simulink model "test44"  (R2015a)
settings: Solver=ode45  StartTime=0.0  StopTime=10.0  RelTol=1e-3
values from neighbouring files (symbols this model uses):
  Ac = A - B*K + L*C    [test3.m]    (also in test4.m; test5.m)
  Bc = -L    [test3.m]    (also in test4.m; test5.m)
  Cc = K    [test3.m]    (also in test4.m; test5.m)
  d1 = m0 + m1 + m2    (= 2.75)    [test3.m]    (also in test4.m; test5.m = 0.00498784618394)
  d2 = (m1/2 + m2) * l1    (= 0.5)    [test3.m]    (also in test4.m; test5.m = 0.00670234055869)
  d3 = m2 * l2/2    (= 0.28125)    [test3.m]    (also in test4.m; test5.m = 0.00902586221044)
  d4 = (m1/3 + m2) * l1^2    (= 0.229166666667)    [test3.m]    (also in test4.m)
  d5 = m2 * l1 * l2/2    (= 0.140625)    [test3.m]    (also in test4.m)
  d6 = m2 * l2^2/3    (= 0.140625)    [test3.m]    (also in test4.m)
  Dc = 0    [test3.m]    (also in test4.m; test5.m)
  f1 = (m1/2 + m2) * l1 * g    (= 4.9)    [test3.m]    (also in test4.m; test5.m = 0.66350669926)
  f2 = m2 * l2 *g/2    (= 2.75625)    [test3.m]    (also in test4.m; test5.m = 0.891162386564)
  r = 0    [test2.m]    (also in test3.m; test4.m; test5.m)
settings Model: Creator=joseg  LastModifiedBy=joseg

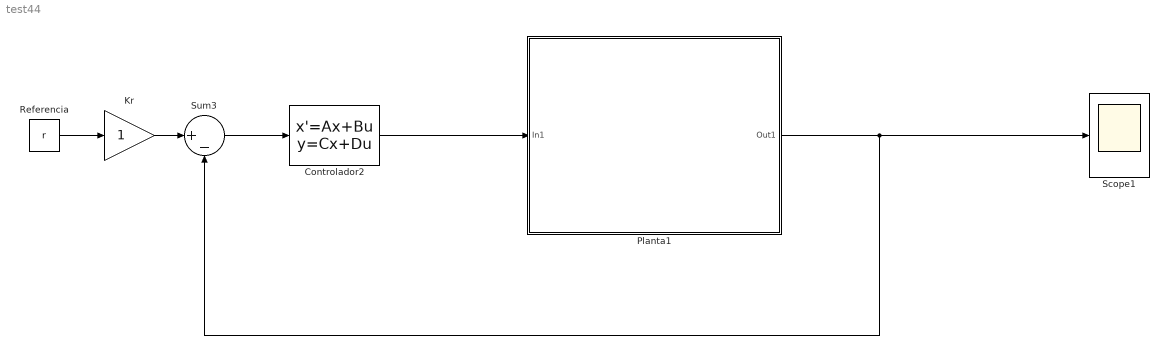
== system test44 ==
  Controlador2 : StateSpace  A=Ac  B=Bc  C=Cc  D=Dc  X0=[0;0;0;0;0;0]
  Kr : Gain
  Planta1 : Subsystem
  Referencia : Constant  Value=r
  Scope1 : Scope
      settings: TimeRange=10  YMin=-21950  YMax=-21350  SaveName=ScopeData2
  Sum3 : Sum  Inputs=|+-
  wires:
  Planta1/1(Out1) -> Sum3/2, Scope1/1
  Sum3/1 -> Controlador2/1
  Kr/1 -> Sum3/1
  Controlador2/1 -> Planta1/1(In1)
  Referencia/1 -> Kr/1

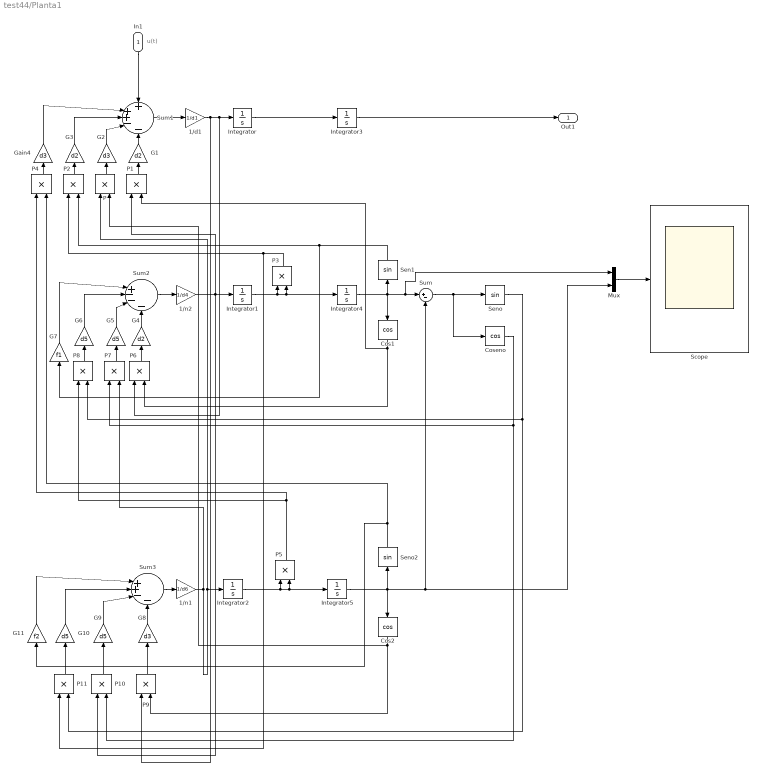
== system test44/Planta1 ==
  note: u(t)
  In1 : Inport
  1/d1 : Gain  Gain=1/d1
  1/n1 : Gain  Gain=1/d6
  1/n2 : Gain  Gain=1/d4
  Cos1 : Trigonometry  Operator=cos
  Cos2 : Trigonometry  Operator=cos
  Coseno : Trigonometry  Operator=cos
  G1 : Gain  Gain=d2
  G{5..6,9..10} (4 alike) : Gain  Gain=d5
  G11 : Gain  Gain=f2
  G2 : Gain  Gain=d3
  G3 : Gain  Gain=d2
  G4 : Gain  Gain=d2
  G7 : Gain  Gain=f1
  G8 : Gain  Gain=d3
  Gain4 : Gain  Gain=d3
  Integrator{,1..3} (4 alike) : Integrator
  Integrator4 : Integrator  InitialCondition=pi
  Integrator5 : Integrator  InitialCondition=pi
  Mux : Mux  Inputs=2
  P{,1..11} (12 alike) : Product
  Scope : Scope
      settings: ShowLegends=on
  Sen1 : Trigonometry
  Seno : Trigonometry
  Seno2 : Trigonometry
  Sum : Sum  Inputs=|+-
  Sum1 : Sum  Inputs=+|++-|-
  Sum2 : Sum  Inputs=||+--|-
  Sum3 : Sum  Inputs=||++-|-
  Out1 : Outport
  wires:
  Integrator/1 -> Integrator3/1
  Integrator1/1 -> P3/1, P3/2, Integrator4/1
  Integrator2/1 -> P5/1, P5/2, Integrator5/1
  Integrator4/1 -> Cos1/1, Sen1/1, Mux/1, Sum/1
  Integrator5/1 -> Cos2/1, Seno2/1, Mux/2, Sum/2
  Sum/1 -> Coseno/1, Seno/1
  Integrator3/1 -> Out1/1
  In1/1 -> Sum1/1
  Sum1/1 -> 1/d1/1
  1/d1/1 -> P9/1, P6/1, Integrator/1
  G1/1 -> Sum1/5
  P1/1 -> G1/1
  Cos1/1 -> P1/2, P6/2
  Sum2/1 -> 1/n2/1
  P/1 -> G2/1
  Cos2/1 -> P9/2, P/2
  G2/1 -> Sum1/4
  Sum3/1 -> 1/n1/1
  G3/1 -> Sum1/3
  P2/1 -> G3/1
  Sen1/1 -> P2/2, G7/1
  P3/1 -> P2/1, P11/1
  P4/1 -> Gain4/1
  Gain4/1 -> Sum1/2
  Seno2/1 -> G11/1, P4/2
  P5/1 -> P8/1, P4/1
  1/n2/1 -> P10/1, Integrator1/1, P1/1
  G4/1 -> Sum2/4
  P6/1 -> G4/1
  G5/1 -> Sum2/3
  P7/1 -> G5/1
  Coseno/1 -> P10/2, P7/1
  P8/1 -> G6/1
  Seno/1 -> P8/2, P11/2
  G6/1 -> Sum2/2
  G7/1 -> Sum2/1
  1/n1/1 -> Integrator2/1, P/1, P7/2
  G8/1 -> Sum3/4
  P9/1 -> G8/1
  G9/1 -> Sum3/3
  P10/1 -> G9/1
  G10/1 -> Sum3/2
  P11/1 -> G10/1
  G11/1 -> Sum3/1
  Mux/1 -> Scope/1
